simulink library "CurrentsLib"  (Simulink 7.7)
settings: Solver=ode45  SolverMode=SingleTasking  StartTime=0.0  StopTime=10.0  RelTol=1e-3
undefined symbols (not defined in the file or in its folder): A, B, diff1, EX, G, gX, PfAHP, PmAHP, PsAHP, Q0, S, T
libraries: CurrentsLib x75, WaveformsLib x11
(part 2 of 2)

== system CurrentsLib/L-type Ca Current , ICaL/h Equil-Eqs Gate/EquilFunct ==
  v : Inport
  caLh_infin2 : CurrentsLib/StateFunctFormIII  SystemSampleTime=-1  T=-20  S=-1/5  B=1  G=1
  s : Outport
  wires:
  v/1 -> caLh_infin2/1
  caLh_infin2/1 -> s/1

== system CurrentsLib/L-type Ca Current , ICaL/h Equil-Eqs Gate/TauFunct ==
  v : Inport
  cah_tau2 : CurrentsLib/caLh_tau  SystemSampleTime=-1
  s : Outport
  wires:
  v/1 -> cah_tau2/1
  cah_tau2/1 -> s/1

== system CurrentsLib/N-type Ca Current, ICaN/h Equil Eqs Gate/EquilFunct ==
  v : Inport
  caNh_infin2 : CurrentsLib/StateFunctFormIII  SystemSampleTime=-1  T=-20  S=-1/5  B=1  G=1
  s : Outport
  wires:
  v/1 -> caNh_infin2/1
  caNh_infin2/1 -> s/1

== system CurrentsLib/N-type Ca Current, ICaN/h Equil Eqs Gate/TauFunct ==
  v : Inport
  cah_tau2 : CurrentsLib/caLh_tau  SystemSampleTime=-1
  s : Outport
  wires:
  v/1 -> cah_tau2/1
  cah_tau2/1 -> s/1

== system CurrentsLib/P-type Ca Current, ICaP/h Equil-Eqs Gate/EquilFunct ==
  v : Inport
  caPh_infin2 : CurrentsLib/StateFunctFormIII  SystemSampleTime=-1  T=-18  S=-1/5.5  B=1  G=1
  s : Outport
  wires:
  v/1 -> caPh_infin2/1
  caPh_infin2/1 -> s/1

== system CurrentsLib/P-type Ca Current, ICaP/h Equil-Eqs Gate/TauFunct ==
  v : Inport
  cah_tau2 : CurrentsLib/caLh_tau  SystemSampleTime=-1
  s : Outport
  wires:
  v/1 -> cah_tau2/1
  cah_tau2/1 -> s/1
